simulink model "car_model"  (R2020a)
settings: Solver=FixedStepAuto  StartTime=0.0  StopTime=120  FixedStep=0.01  RelTol=1e-3
values from neighbouring files (symbols this model uses):
  A = 2.18    [car_startup.m]
  brake_force = 7500    [car_startup.m]
  cx = 0.3    [car_startup.m]
  eff = 0.9    [car_startup.m]
  f0 = 0.01    [car_startup.m]
  g = 9.81    [car_startup.m]
  ibi = [3.31 1.91 1.31 0.97 0.81]    [car_startup.m]
  ig = 4.53    [car_startup.m]
  m = 955    [car_startup.m]
  rd = 0.360    (= 0.36)    [car_startup.m]
  start_speed = 0    [car_startup.m]
  torque_curve_f = polyfit(csv_data(:,1), csv_data(:,2), 2)    [car_startup.m]
libraries: simulink x4, SignalEditorBlockLib x1
settings Model: Creator=cp  LastModifiedBy=cp
settings DataIOCC: ReturnWorkspaceOutputs=off  ReturnWorkspaceOutputsName=car
settings OptimizationCC: BlockReduction=off  DefaultParameterBehavior=Inlined  BufferReuse=off

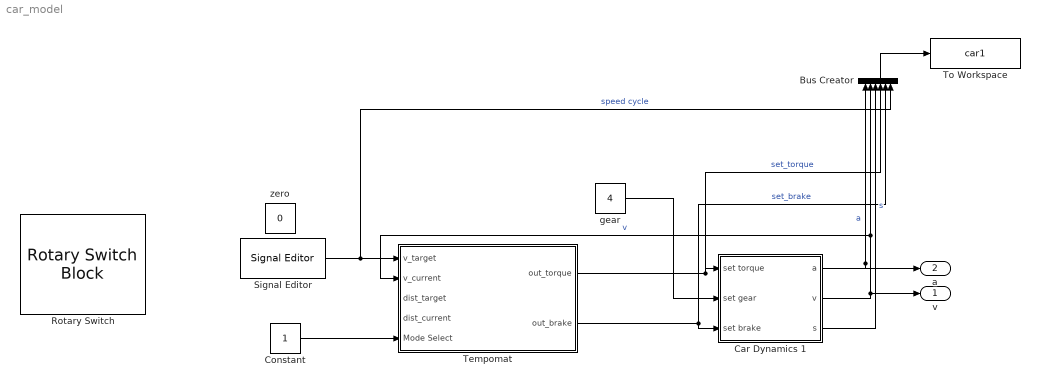
== system car_model ==
  Bus Creator : BusCreator  Inputs=6
  Car Dynamics 1 : Subsystem
  Constant : Constant
  Rotary Switch : RotarySwitchBlock
      settings: Values={{'1', '2', '3', '4', '5'}, [1 2 3 4 5]}
  Signal Editor : SignalEditorBlockLib/Signal Editor  FileName=cycle1.mat  ActiveScenario=Scenario1  ActiveSignal=Signal 1  IsBus=off  OutputBusObjectStr=Bus: BusObject  SampleTime=0  Interpolate=off  ZeroCross=off  OutputAfterFinalValue=Holding final value  Unit=inherit  PreserveSignalName=on
  Tempomat : Subsystem
  To Workspace : ToWorkspace  VariableName=car1  SaveFormat=Timeseries  SampleTime=-1
  gear : Constant  Value=4
  v : Outport
  a : Outport  Port=2
  zero : Constant  IOType=siggen  Value=0
  wires:
  Car Dynamics 1/1(a) -> Bus Creator/1, a/1  "a"
  Car Dynamics 1/2(v) -> Tempomat/2(v_current), Bus Creator/2, v/1  "v"
  Tempomat/1(out_torque) -> Car Dynamics 1/1(set torque), Bus Creator/4  "set_torque"
  gear/1 -> Car Dynamics 1/2(set gear)
  Tempomat/2(out_brake) -> Car Dynamics 1/3(set brake), Bus Creator/5  "set_brake"
  Signal Editor/1 -> Bus Creator/6, Tempomat/1(v_target)  "speed cycle"
  Bus Creator/1 -> To Workspace/1
  Car Dynamics 1/3(s) -> Bus Creator/3  "s"
  Constant/1 -> Tempomat/5(Mode Select)

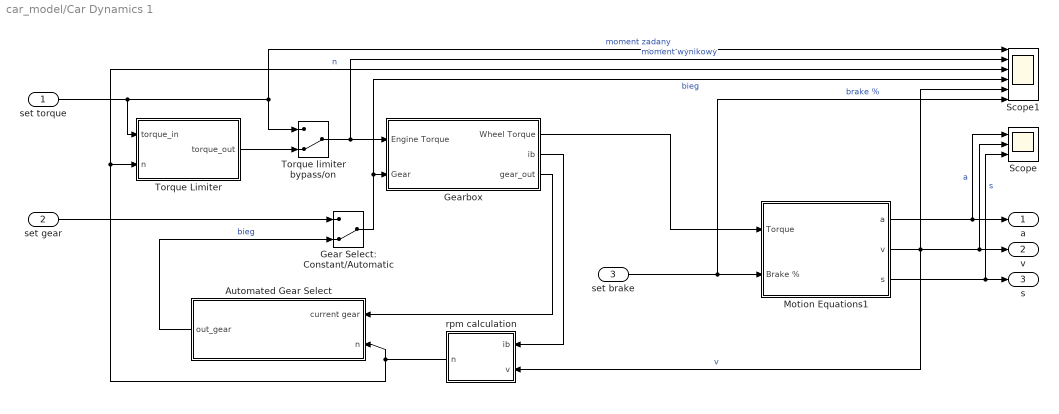
== system car_model/Car Dynamics 1 ==
  set torque : Inport
  set gear : Inport  Port=2
  set brake : Inport  Port=3
  Automated Gear Select : Subsystem
  Gear Select: Constant/Automatic : ManualSwitch  CurrentSetting=0
  Gearbox : Subsystem
  Motion Equations1 : Subsystem  VariantControl=Choice
  Scope : Scope  NumInputPorts=3
  Scope1 : Scope  NumInputPorts=6
  Torque Limiter : Subsystem
  Torque limiter bypass/on : ManualSwitch  CurrentSetting=0
  rpm calculation : Subsystem
  a : Outport
  v : Outport  Port=2
  s : Outport  Port=3
  wires:
  set torque/1 -> Torque limiter bypass/on/1, Scope1/1, Torque Limiter/1(torque_in)  "moment zadany"
  Gearbox/2(ib) -> rpm calculation/1(ib)
  Gear Select: Constant/Automatic/1 -> Scope1/4, Gearbox/2(Gear)  "bieg"
  Automated Gear Select/1(out_gear) -> Gear Select: Constant/Automatic/2  "bieg"
  set gear/1 -> Gear Select: Constant/Automatic/1
  Gearbox/3(gear_out) -> Automated Gear Select/1(current gear)
  rpm calculation/1(n) -> Scope1/3, Torque Limiter/2(n), Automated Gear Select/2(n)  "n"
  Torque limiter bypass/on/1 -> Scope1/2, Gearbox/1(Engine Torque)  "moment wynikowy"
  Torque Limiter/1(torque_out) -> Torque limiter bypass/on/2
  set brake/1 -> Motion Equations1/2(Brake %), Scope1/6  "brake %"
  Gearbox/1(Wheel Torque) -> Motion Equations1/1(Torque)
  Motion Equations1/1(a) -> Scope/1, a/1  "a"
  Motion Equations1/2(v) -> Scope/2, v/1, Scope1/5, rpm calculation/2(v)  "v"
  Motion Equations1/3(s) -> Scope/3, s/1  "s"

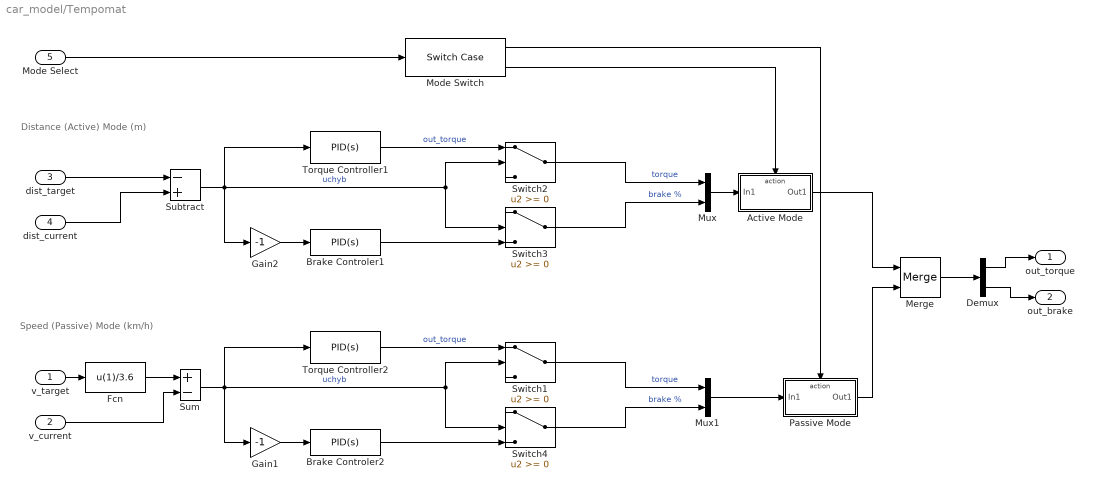
== system car_model/Tempomat ==
  note: Distance (Active) Mode (m)
  note: Speed (Passive) Mode (km/h)
  v_target : Inport
  v_current : Inport  Port=2
  dist_target : Inport  Port=3
  dist_current : Inport  Port=4
  Mode Select : Inport  Port=5
  Active Mode : Subsystem  TreatAsAtomicUnit=on
  Brake Controler1 : simulink/Continuous/PID Controller  Controller=PID  Form=Parallel  TimeDomain=Continuous-time  UseExternalTs=off  SampleTime=-1  IntegratorMethod=Forward Euler  FilterMethod=Forward Euler  ControllerParametersSource=internal  P=5  I=0.5  D=0  UseFilter=on  N=100  TunerSelectOption=Transfer Function Based (PID Tuner App)  InitialConditionSource=internal  InitialConditionForIntegrator=0  InitialConditionForFilter=0  DifferentiatorICPrevScaledInput=0  ExternalReset=none  TrackingMode=off  Kt=1  LimitOutput=on  UpperSaturationLimit=100  LowerSaturationLimit=0  LinearizeAsGain=on  AntiWindupMode=none  Kb=1  POutMin=[]  POutMax=[]  IOutMin=[]  IOutMax=[]  DOutMin=[]  DOutMax=[]  NOutMin=[]  NOutMax=[]  SumOutMin=[]  SumOutMax=[]  SaturationOutMin=[]  SaturationOutMax=[]  PParamMin=[]  PParamMax=[]  IParamMin=[]  IParamMax=[]  DParamMin=[]  DParamMax=[]  NParamMin=[]  NParamMax=[]  KbParamMin=[]  KbParamMax=[]  KtParamMin=[]  KtParamMax=[]  KbOutMin=[]  KbOutMax=[]  KtOutMin=[]  KtOutMax=[]  IntegratorOutMin=[]  IntegratorOutMax=[]  FilterOutMin=[]  FilterOutMax=[]  SumI1OutMin=[]  SumI1OutMax=[]  SumI2OutMin=[]  SumI2OutMax=[]  SumI3OutMin=[]  SumI3OutMax=[]  SumI4OutMin=[]  SumI4OutMax=[]  SumDOutMin=[]  SumDOutMax=[]  DifferentiatorOutMin=[]  DifferentiatorOutMax=[]  FilterDiffOutCoefMin=[]  FilterDiffOutCoefMax=[]  ReciprocalOutMin=[]  ReciprocalOutMax=[]  SumDenOutMin=[]  SumDenOutMax=[]  SumNumOutMin=[]  SumNumOutMax=[]  DivideOutMin=[]  DivideOutMax=[]  UdiffTsProdOutMin=[]  UdiffTsProdOutMax=[]  NTsProdOutMin=[]  NTsProdOutMax=[]  UintegralTsProdOutMin=[]  UintegralTsProdOutMax=[]  UngainTsProdOutMin=[]  UngainTsProdOutMax=[]  IntegratorContinuousStateAttributes=''  IntegratorStateMustResolveToSignalObject=off  IntegratorRTWStateStorageClass=Auto  FilterContinuousStateAttributes=''  FilterStateMustResolveToSignalObject=off  FilterRTWStateStorageClass=Auto  ParallelPVariant=InternalParameters  IdealPVariant=Disabled  IVariant=InternalParameters  DVariant=InternalParameters  IntegratorVariant=Continuous  SatVariant=Enabled  AWVariant=Passthrough  PCopyVariant=Disabled  TRVariant=Disabled  FdbkBlocksVariant=Forward  IdealPFdbkVariant=Disabled  SatFdbkVariant=Disabled  DerivativeFilterVariant=ContFilter  NVariant=InternalParameters  NCopyVariant=Disabled  FilterICVariant=InternalICsFilter  IntegratorICVariant=InternalICs  ExternalResetVariant=Disabled  TRSumVariant=Passthrough  SumFdbkVariant=Disabled  SumVariant=Sum_PID  TsampFilterVariant=InternalTs  TsampNgainVariant=Passthrough  TsampIntegralVariant=Passthrough
  Brake Controler2 : simulink/Continuous/PID Controller  Controller=PID  Form=Parallel  TimeDomain=Continuous-time  UseExternalTs=off  SampleTime=-1  IntegratorMethod=Forward Euler  FilterMethod=Forward Euler  ControllerParametersSource=internal  P=5  I=0.5  D=0  UseFilter=on  N=100  TunerSelectOption=Transfer Function Based (PID Tuner App)  InitialConditionSource=internal  InitialConditionForIntegrator=0  InitialConditionForFilter=0  DifferentiatorICPrevScaledInput=0  ExternalReset=none  TrackingMode=off  Kt=1  LimitOutput=on  UpperSaturationLimit=100  LowerSaturationLimit=0  LinearizeAsGain=on  AntiWindupMode=none  Kb=1  POutMin=[]  POutMax=[]  IOutMin=[]  IOutMax=[]  DOutMin=[]  DOutMax=[]  NOutMin=[]  NOutMax=[]  SumOutMin=[]  SumOutMax=[]  SaturationOutMin=[]  SaturationOutMax=[]  PParamMin=[]  PParamMax=[]  IParamMin=[]  IParamMax=[]  DParamMin=[]  DParamMax=[]  NParamMin=[]  NParamMax=[]  KbParamMin=[]  KbParamMax=[]  KtParamMin=[]  KtParamMax=[]  KbOutMin=[]  KbOutMax=[]  KtOutMin=[]  KtOutMax=[]  IntegratorOutMin=[]  IntegratorOutMax=[]  FilterOutMin=[]  FilterOutMax=[]  SumI1OutMin=[]  SumI1OutMax=[]  SumI2OutMin=[]  SumI2OutMax=[]  SumI3OutMin=[]  SumI3OutMax=[]  SumI4OutMin=[]  SumI4OutMax=[]  SumDOutMin=[]  SumDOutMax=[]  DifferentiatorOutMin=[]  DifferentiatorOutMax=[]  FilterDiffOutCoefMin=[]  FilterDiffOutCoefMax=[]  ReciprocalOutMin=[]  ReciprocalOutMax=[]  SumDenOutMin=[]  SumDenOutMax=[]  SumNumOutMin=[]  SumNumOutMax=[]  DivideOutMin=[]  DivideOutMax=[]  UdiffTsProdOutMin=[]  UdiffTsProdOutMax=[]  NTsProdOutMin=[]  NTsProdOutMax=[]  UintegralTsProdOutMin=[]  UintegralTsProdOutMax=[]  UngainTsProdOutMin=[]  UngainTsProdOutMax=[]  IntegratorContinuousStateAttributes=''  IntegratorStateMustResolveToSignalObject=off  IntegratorRTWStateStorageClass=Auto  FilterContinuousStateAttributes=''  FilterStateMustResolveToSignalObject=off  FilterRTWStateStorageClass=Auto  ParallelPVariant=InternalParameters  IdealPVariant=Disabled  IVariant=InternalParameters  DVariant=InternalParameters  IntegratorVariant=Continuous  SatVariant=Enabled  AWVariant=Passthrough  PCopyVariant=Disabled  TRVariant=Disabled  FdbkBlocksVariant=Forward  IdealPFdbkVariant=Disabled  SatFdbkVariant=Disabled  DerivativeFilterVariant=ContFilter  NVariant=InternalParameters  NCopyVariant=Disabled  FilterICVariant=InternalICsFilter  IntegratorICVariant=InternalICs  ExternalResetVariant=Disabled  TRSumVariant=Passthrough  SumFdbkVariant=Disabled  SumVariant=Sum_PID  TsampFilterVariant=InternalTs  TsampNgainVariant=Passthrough  TsampIntegralVariant=Passthrough
  Demux : Demux  Outputs=2
  Fcn : Fcn  Expr=u(1)/3.6
  Gain1 : Gain  Gain=-1
  Gain2 : Gain  Gain=-1
  Merge : Merge
  Mode Switch : SwitchCase
  Mux : Mux  Inputs=2
  Mux1 : Mux  Inputs=2
  Passive Mode : Subsystem  TreatAsAtomicUnit=on
  Subtract : Sum  Inputs=-+
  Sum : Sum  Inputs=+-
  Switch{1..4} (4 alike) : Switch
  Torque Controller1 : simulink/Continuous/PID Controller  Controller=PID  Form=Parallel  TimeDomain=Continuous-time  UseExternalTs=off  SampleTime=-1  IntegratorMethod=Forward Euler  FilterMethod=Forward Euler  ControllerParametersSource=internal  P=63.1289554713546  I=0  D=0  UseFilter=on  N=0.822866017947126  TunerSelectOption=Transfer Function Based (PID Tuner App)  InitialConditionSource=internal  InitialConditionForIntegrator=0  InitialConditionForFilter=0  DifferentiatorICPrevScaledInput=0  ExternalReset=none  TrackingMode=off  Kt=1  LimitOutput=on  UpperSaturationLimit=148  LowerSaturationLimit=0  LinearizeAsGain=on  AntiWindupMode=none  Kb=1  POutMin=[]  POutMax=[]  IOutMin=[]  IOutMax=[]  DOutMin=[]  DOutMax=[]  NOutMin=[]  NOutMax=[]  SumOutMin=[]  SumOutMax=[]  SaturationOutMin=[]  SaturationOutMax=[]  PParamMin=[]  PParamMax=[]  IParamMin=[]  IParamMax=[]  DParamMin=[]  DParamMax=[]  NParamMin=[]  NParamMax=[]  KbParamMin=[]  KbParamMax=[]  KtParamMin=[]  KtParamMax=[]  KbOutMin=[]  KbOutMax=[]  KtOutMin=[]  KtOutMax=[]  IntegratorOutMin=[]  IntegratorOutMax=[]  FilterOutMin=[]  FilterOutMax=[]  SumI1OutMin=[]  SumI1OutMax=[]  SumI2OutMin=[]  SumI2OutMax=[]  SumI3OutMin=[]  SumI3OutMax=[]  SumI4OutMin=[]  SumI4OutMax=[]  SumDOutMin=[]  SumDOutMax=[]  DifferentiatorOutMin=[]  DifferentiatorOutMax=[]  FilterDiffOutCoefMin=[]  FilterDiffOutCoefMax=[]  ReciprocalOutMin=[]  ReciprocalOutMax=[]  SumDenOutMin=[]  SumDenOutMax=[]  SumNumOutMin=[]  SumNumOutMax=[]  DivideOutMin=[]  DivideOutMax=[]  UdiffTsProdOutMin=[]  UdiffTsProdOutMax=[]  NTsProdOutMin=[]  NTsProdOutMax=[]  UintegralTsProdOutMin=[]  UintegralTsProdOutMax=[]  UngainTsProdOutMin=[]  UngainTsProdOutMax=[]  IntegratorContinuousStateAttributes=''  IntegratorStateMustResolveToSignalObject=off  IntegratorRTWStateStorageClass=Auto  FilterContinuousStateAttributes=''  FilterStateMustResolveToSignalObject=off  FilterRTWStateStorageClass=Auto  ParallelPVariant=InternalParameters  IdealPVariant=Disabled  IVariant=InternalParameters  DVariant=InternalParameters  IntegratorVariant=Continuous  SatVariant=Enabled  AWVariant=Passthrough  PCopyVariant=Disabled  TRVariant=Disabled  FdbkBlocksVariant=Forward  IdealPFdbkVariant=Disabled  SatFdbkVariant=Disabled  DerivativeFilterVariant=ContFilter  NVariant=InternalParameters  NCopyVariant=Disabled  FilterICVariant=InternalICsFilter  IntegratorICVariant=InternalICs  ExternalResetVariant=Disabled  TRSumVariant=Passthrough  SumFdbkVariant=Disabled  SumVariant=Sum_PID  TsampFilterVariant=InternalTs  TsampNgainVariant=Passthrough  TsampIntegralVariant=Passthrough
  Torque Controller2 : simulink/Continuous/PID Controller  Controller=PID  Form=Parallel  TimeDomain=Continuous-time  UseExternalTs=off  SampleTime=-1  IntegratorMethod=Forward Euler  FilterMethod=Forward Euler  ControllerParametersSource=internal  P=63.1289554713546  I=0  D=0  UseFilter=on  N=0.822866017947126  TunerSelectOption=Transfer Function Based (PID Tuner App)  InitialConditionSource=internal  InitialConditionForIntegrator=0  InitialConditionForFilter=0  DifferentiatorICPrevScaledInput=0  ExternalReset=none  TrackingMode=off  Kt=1  LimitOutput=on  UpperSaturationLimit=148  LowerSaturationLimit=0  LinearizeAsGain=on  AntiWindupMode=none  Kb=1  POutMin=[]  POutMax=[]  IOutMin=[]  IOutMax=[]  DOutMin=[]  DOutMax=[]  NOutMin=[]  NOutMax=[]  SumOutMin=[]  SumOutMax=[]  SaturationOutMin=[]  SaturationOutMax=[]  PParamMin=[]  PParamMax=[]  IParamMin=[]  IParamMax=[]  DParamMin=[]  DParamMax=[]  NParamMin=[]  NParamMax=[]  KbParamMin=[]  KbParamMax=[]  KtParamMin=[]  KtParamMax=[]  KbOutMin=[]  KbOutMax=[]  KtOutMin=[]  KtOutMax=[]  IntegratorOutMin=[]  IntegratorOutMax=[]  FilterOutMin=[]  FilterOutMax=[]  SumI1OutMin=[]  SumI1OutMax=[]  SumI2OutMin=[]  SumI2OutMax=[]  SumI3OutMin=[]  SumI3OutMax=[]  SumI4OutMin=[]  SumI4OutMax=[]  SumDOutMin=[]  SumDOutMax=[]  DifferentiatorOutMin=[]  DifferentiatorOutMax=[]  FilterDiffOutCoefMin=[]  FilterDiffOutCoefMax=[]  ReciprocalOutMin=[]  ReciprocalOutMax=[]  SumDenOutMin=[]  SumDenOutMax=[]  SumNumOutMin=[]  SumNumOutMax=[]  DivideOutMin=[]  DivideOutMax=[]  UdiffTsProdOutMin=[]  UdiffTsProdOutMax=[]  NTsProdOutMin=[]  NTsProdOutMax=[]  UintegralTsProdOutMin=[]  UintegralTsProdOutMax=[]  UngainTsProdOutMin=[]  UngainTsProdOutMax=[]  IntegratorContinuousStateAttributes=''  IntegratorStateMustResolveToSignalObject=off  IntegratorRTWStateStorageClass=Auto  FilterContinuousStateAttributes=''  FilterStateMustResolveToSignalObject=off  FilterRTWStateStorageClass=Auto  ParallelPVariant=InternalParameters  IdealPVariant=Disabled  IVariant=InternalParameters  DVariant=InternalParameters  IntegratorVariant=Continuous  SatVariant=Enabled  AWVariant=Passthrough  PCopyVariant=Disabled  TRVariant=Disabled  FdbkBlocksVariant=Forward  IdealPFdbkVariant=Disabled  SatFdbkVariant=Disabled  DerivativeFilterVariant=ContFilter  NVariant=InternalParameters  NCopyVariant=Disabled  FilterICVariant=InternalICsFilter  IntegratorICVariant=InternalICs  ExternalResetVariant=Disabled  TRSumVariant=Passthrough  SumFdbkVariant=Disabled  SumVariant=Sum_PID  TsampFilterVariant=InternalTs  TsampNgainVariant=Passthrough  TsampIntegralVariant=Passthrough
  out_torque : Outport
  out_brake : Outport  Port=2
  wires:
  v_target/1 -> Fcn/1
  Fcn/1 -> Sum/1
  v_current/1 -> Sum/2
  Gain1/1 -> Brake Controler2/1
  Brake Controler2/1 -> Switch4/3
  Switch1/1 -> Mux1/1  "torque"
  Switch4/1 -> Mux1/2  "brake %"
  Torque Controller2/1 -> Switch1/1  "out_torque"
  Sum/1 -> Gain1/1, Switch1/2, Switch4/2, Torque Controller2/1  "uchyb"
  Gain2/1 -> Brake Controler1/1
  Switch3/1 -> Mux/2  "brake %"
  Torque Controller1/1 -> Switch2/1  "out_torque"
  Brake Controler1/1 -> Switch3/3
  Subtract/1 -> Gain2/1, Switch2/2, Switch3/2, Torque Controller1/1  "uchyb"
  Switch2/1 -> Mux/1  "torque"
  Mode Select/1 -> Mode Switch/1
  Mode Switch/2 -> Active Mode/Action
  Mode Switch/1 -> Passive Mode/Action
  Mux/1 -> Active Mode/1(In1)
  Active Mode/1(Out1) -> Merge/1
  Passive Mode/1(Out1) -> Merge/2
  Merge/1 -> Demux/1
  dist_target/1 -> Subtract/1
  dist_current/1 -> Subtract/2
  Demux/1 -> out_torque/1
  Demux/2 -> out_brake/1
  Mux1/1 -> Passive Mode/1(In1)

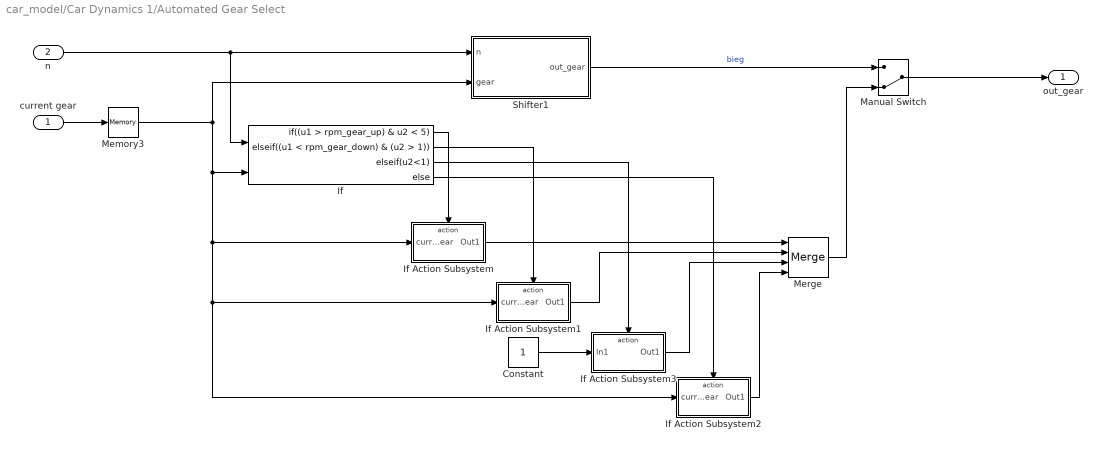
== system car_model/Car Dynamics 1/Automated Gear Select ==
  current gear : Inport
  n : Inport  Port=2
  Constant : Constant
  If : If  NumInputs=2  IfExpression=(u1 > rpm_gear_up) & u2 < 5  ElseIfExpressions=(u1 < rpm_gear_down) & (u2 > 1), u2<1
  If Action Subsystem : Subsystem  TreatAsAtomicUnit=on
  If Action Subsystem1 : Subsystem  TreatAsAtomicUnit=on
  If Action Subsystem2 : Subsystem  TreatAsAtomicUnit=on
  If Action Subsystem3 : Subsystem  TreatAsAtomicUnit=on
  Manual Switch : ManualSwitch  CurrentSetting=0
  Memory3 : Memory
  Merge : Merge  Inputs=4
  Shifter1 : MATLAB Function  TreatAsAtomicUnit=on
  out_gear : Outport
  wires:
  current gear/1 -> Memory3/1
  Memory3/1 -> Shifter1/2(gear), If Action Subsystem2/1(current gear), If Action Subsystem1/1(current gear), If Action Subsystem/1(current gear), If/2
  n/1 -> If/1, Shifter1/1(n)
  If/1 -> If Action Subsystem/Action
  If/2 -> If Action Subsystem1/Action
  If/4 -> If Action Subsystem2/Action
  If Action Subsystem/1(Out1) -> Merge/1
  If Action Subsystem1/1(Out1) -> Merge/2
  If Action Subsystem2/1(Out1) -> Merge/4
  Shifter1/1(out_gear) -> Manual Switch/1  "bieg"
  Manual Switch/1 -> out_gear/1
  Merge/1 -> Manual Switch/2
  If/3 -> If Action Subsystem3/Action
  If Action Subsystem3/1(Out1) -> Merge/3
  Constant/1 -> If Action Subsystem3/1(In1)

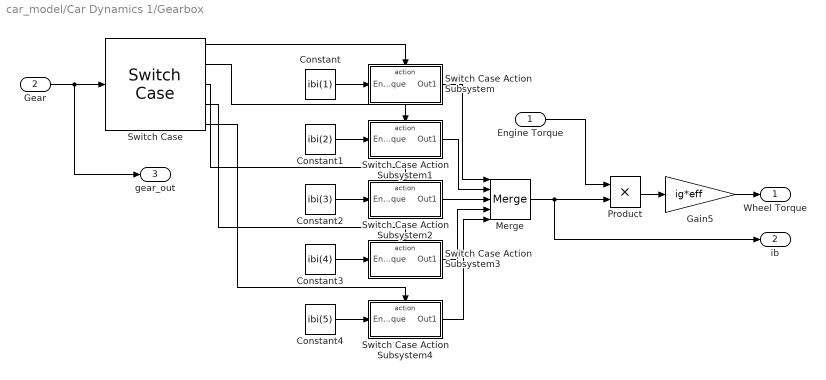
== system car_model/Car Dynamics 1/Gearbox ==
  Engine Torque : Inport
  Gear : Inport  Port=2
  Constant : Constant  Value=ibi(1)
  Constant1 : Constant  Value=ibi(2)
  Constant2 : Constant  Value=ibi(3)
  Constant3 : Constant  Value=ibi(4)
  Constant4 : Constant  Value=ibi(5)
  Gain5 : Gain  Gain=ig*eff
  Merge : Merge  Inputs=5
  Product : Product
  Switch Case : SwitchCase  CaseConditions={[0,1],2,3,4,5}  ShowDefaultCase=off
  Switch Case Action Subsystem : Subsystem  TreatAsAtomicUnit=on
  Switch Case Action Subsystem1 : Subsystem  TreatAsAtomicUnit=on
  Switch Case Action Subsystem2 : Subsystem  TreatAsAtomicUnit=on
  Switch Case Action Subsystem3 : Subsystem  TreatAsAtomicUnit=on
  Switch Case Action Subsystem4 : Subsystem  TreatAsAtomicUnit=on
  Wheel Torque : Outport
  ib : Outport  Port=2
  gear_out : Outport  Port=3
  wires:
  Switch Case/1 -> Switch Case Action Subsystem/Action
  Switch Case/2 -> Switch Case Action Subsystem1/Action
  Switch Case/3 -> Switch Case Action Subsystem2/Action
  Switch Case/4 -> Switch Case Action Subsystem3/Action
  Switch Case/5 -> Switch Case Action Subsystem4/Action
  Constant1/1 -> Switch Case Action Subsystem1/1(Engine Torque)
  Constant/1 -> Switch Case Action Subsystem/1(Engine Torque)
  Switch Case Action Subsystem/1(Out1) -> Merge/1
  Switch Case Action Subsystem1/1(Out1) -> Merge/2
  Switch Case Action Subsystem2/1(Out1) -> Merge/3
  Switch Case Action Subsystem3/1(Out1) -> Merge/4
  Switch Case Action Subsystem4/1(Out1) -> Merge/5
  Gain5/1 -> Wheel Torque/1
  Gear/1 -> gear_out/1, Switch Case/1
  Merge/1 -> ib/1, Product/2
  Product/1 -> Gain5/1
  Engine Torque/1 -> Product/1
  Constant2/1 -> Switch Case Action Subsystem2/1(Engine Torque)
  Constant3/1 -> Switch Case Action Subsystem3/1(Engine Torque)
  Constant4/1 -> Switch Case Action Subsystem4/1(Engine Torque)

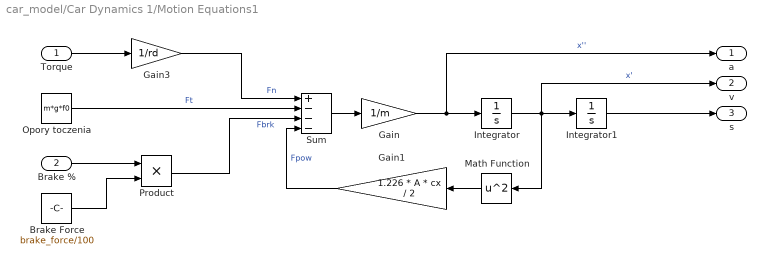
== system car_model/Car Dynamics 1/Motion Equations1 ==
  Torque : Inport
  Brake % : Inport  Port=2
  Brake Force : Constant  Value=brake_force/100
  Gain : Gain  Gain=1/m
  Gain1 : Gain  Gain=1.226 * A * cx / 2
  Gain3 : Gain  Gain=1/rd
  Integrator : Integrator  InitialCondition=start_speed
  Integrator1 : Integrator
  Math Function : Math  Operator=square  SaturateOnIntegerOverflow=on
  Opory toczenia : Constant  Value=m*g*f0
  Product : Product
  Sum : Sum  Inputs=+---
  a : Outport
  v : Outport  Port=2
  s : Outport  Port=3
  wires:
  Integrator1/1 -> s/1
  Sum/1 -> Gain/1
  Math Function/1 -> Gain1/1
  Gain/1 -> a/1, Integrator/1  "x''"
  Integrator/1 -> v/1, Math Function/1, Integrator1/1  "x'"
  Gain1/1 -> Sum/4  "Fpow"
  Opory toczenia/1 -> Sum/2  "Ft"
  Torque/1 -> Gain3/1
  Gain3/1 -> Sum/1  "Fn"
  Brake Force/1 -> Product/2
  Brake %/1 -> Product/1
  Product/1 -> Sum/3  "Fbrk"

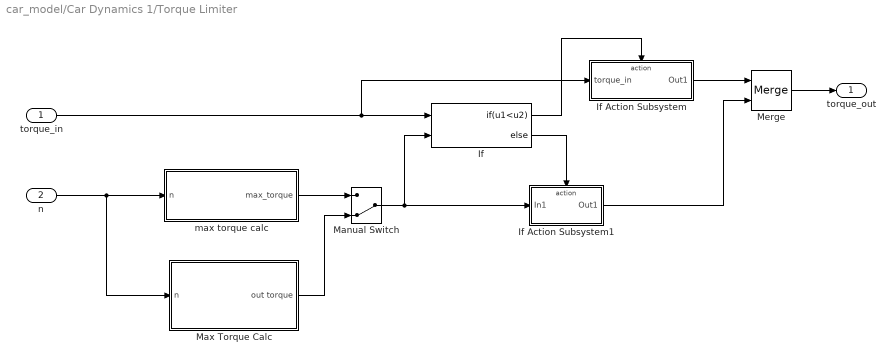
== system car_model/Car Dynamics 1/Torque Limiter ==
  torque_in : Inport
  n : Inport  Port=2
  If : If  NumInputs=2  IfExpression=u1<u2
  If Action Subsystem : Subsystem  TreatAsAtomicUnit=on
  If Action Subsystem1 : Subsystem  TreatAsAtomicUnit=on
  Manual Switch : ManualSwitch  CurrentSetting=0
  Max Torque Calc : Subsystem
  Merge : Merge
  max torque calc : MATLAB Function  TreatAsAtomicUnit=on
  torque_out : Outport
  wires:
  n/1 -> Max Torque Calc/1(n), max torque calc/1(n)
  torque_in/1 -> If Action Subsystem/1(torque_in), If/1
  If/1 -> If Action Subsystem/Action
  Merge/1 -> torque_out/1
  If Action Subsystem/1(Out1) -> Merge/1
  If/2 -> If Action Subsystem1/Action
  If Action Subsystem1/1(Out1) -> Merge/2
  Manual Switch/1 -> If Action Subsystem1/1(In1), If/2
  max torque calc/1(max_torque) -> Manual Switch/1
  Max Torque Calc/1(out torque) -> Manual Switch/2

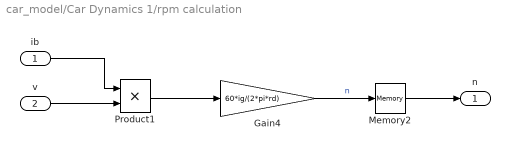
== system car_model/Car Dynamics 1/rpm calculation ==
  ib : Inport
  v : Inport  Port=2
  Gain4 : Gain  Gain=60*ig/(2*pi*rd)
  Memory2 : Memory
  Product1 : Product
  n : Outport
  wires:
  v/1 -> Product1/2
  Memory2/1 -> n/1
  Product1/1 -> Gain4/1
  Gain4/1 -> Memory2/1  "n"
  ib/1 -> Product1/1

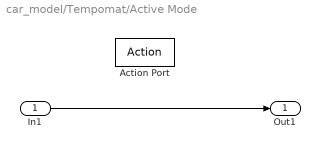
== system car_model/Tempomat/Active Mode ==
  In1 : Inport
  Action Port : ActionPort  ActionPortLabel=default:
  Out1 : Outport
  wires:
  In1/1 -> Out1/1

== system car_model/Tempomat/Passive Mode ==
  In1 : Inport
  Action Port : ActionPort  ActionPortLabel=case [ 1 ]:
  Out1 : Outport
  wires:
  In1/1 -> Out1/1

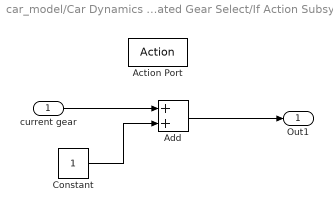
== system car_model/Car Dynamics 1/Automated Gear Select/If Action Subsystem ==
  current gear : Inport
  Action Port : ActionPort  ActionPortLabel=if((u1 > rpm_gear_up) & u2 < 5)
  Add : Sum
  Constant : Constant
  Out1 : Outport
  wires:
  current gear/1 -> Add/1
  Add/1 -> Out1/1
  Constant/1 -> Add/2

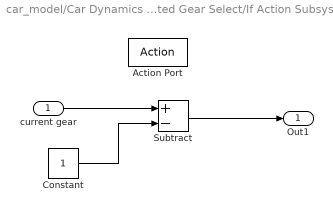
== system car_model/Car Dynamics 1/Automated Gear Select/If Action Subsystem1 ==
  current gear : Inport
  Action Port : ActionPort  ActionPortLabel=elseif((u1 < rpm_gear_down) & (u2 > 1))
  Constant : Constant
  Subtract : Sum  Inputs=+-
  Out1 : Outport
  wires:
  current gear/1 -> Subtract/1
  Subtract/1 -> Out1/1
  Constant/1 -> Subtract/2

== system car_model/Car Dynamics 1/Automated Gear Select/If Action Subsystem2 ==
  current gear : Inport
  Action Port : ActionPort  ActionPortLabel=else
  Out1 : Outport
  wires:
  current gear/1 -> Out1/1

== system car_model/Car Dynamics 1/Automated Gear Select/If Action Subsystem3 ==
  In1 : Inport
  Action Port : ActionPort  ActionPortLabel=elseif( u2<1)
  Out1 : Outport
  wires:
  In1/1 -> Out1/1

== system car_model/Car Dynamics 1/Gearbox/Switch Case Action Subsystem ==
  Engine Torque : Inport
  Action Port : ActionPort  ActionPortLabel=case [ 0 1 ]:
  Out1 : Outport
  wires:
  Engine Torque/1 -> Out1/1

== system car_model/Car Dynamics 1/Gearbox/Switch Case Action Subsystem1 ==
  Engine Torque : Inport
  Action Port : ActionPort  ActionPortLabel=case [ 2 ]:
  Out1 : Outport
  wires:
  Engine Torque/1 -> Out1/1

== system car_model/Car Dynamics 1/Gearbox/Switch Case Action Subsystem2 ==
  Engine Torque : Inport
  Action Port : ActionPort  ActionPortLabel=case [ 3 ]:
  Out1 : Outport
  wires:
  Engine Torque/1 -> Out1/1

== system car_model/Car Dynamics 1/Gearbox/Switch Case Action Subsystem3 ==
  Engine Torque : Inport
  Action Port : ActionPort  ActionPortLabel=case [ 4 ]:
  Out1 : Outport
  wires:
  Engine Torque/1 -> Out1/1

== system car_model/Car Dynamics 1/Gearbox/Switch Case Action Subsystem4 ==
  Engine Torque : Inport
  Action Port : ActionPort  ActionPortLabel=case [ 5 ]:
  Out1 : Outport
  wires:
  Engine Torque/1 -> Out1/1

== system car_model/Car Dynamics 1/Torque Limiter/If Action Subsystem ==
  torque_in : Inport
  Action Port : ActionPort  ActionPortLabel=if(u1<u2)
  Out1 : Outport
  wires:
  torque_in/1 -> Out1/1

== system car_model/Car Dynamics 1/Torque Limiter/If Action Subsystem1 ==
  In1 : Inport
  Action Port : ActionPort  ActionPortLabel=else
  Out1 : Outport
  wires:
  In1/1 -> Out1/1

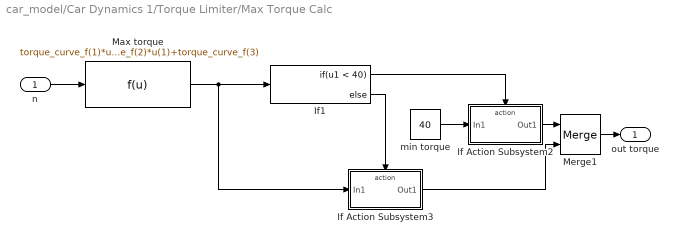
== system car_model/Car Dynamics 1/Torque Limiter/Max Torque Calc ==
  n : Inport
  If Action Subsystem2 : Subsystem  TreatAsAtomicUnit=on
  If Action Subsystem3 : Subsystem  TreatAsAtomicUnit=on
  If1 : If  IfExpression=u1 < 40
  Max torque : Fcn  Expr=torque_curve_f(1)*u(1)^2 + torque_curve_f(2)*u(1)+torque_curve_f(3)
  Merge1 : Merge
  min torque : Constant  Value=40
  out torque : Outport
  wires:
  n/1 -> Max torque/1
  Merge1/1 -> out torque/1
  If Action Subsystem2/1(Out1) -> Merge1/1
  If1/1 -> If Action Subsystem2/Action
  Max torque/1 -> If Action Subsystem3/1(In1), If1/1
  min torque/1 -> If Action Subsystem2/1(In1)
  If Action Subsystem3/1(Out1) -> Merge1/2
  If1/2 -> If Action Subsystem3/Action

== system car_model/Car Dynamics 1/Torque Limiter/Max Torque Calc/If Action Subsystem2 ==
  In1 : Inport
  Action Port : ActionPort  ActionPortLabel=if(u1 < 40)
  Out1 : Outport
  wires:
  In1/1 -> Out1/1

== system car_model/Car Dynamics 1/Torque Limiter/Max Torque Calc/If Action Subsystem3 ==
  In1 : Inport
  Action Port : ActionPort  ActionPortLabel=else
  Out1 : Outport
  wires:
  In1/1 -> Out1/1

== matlab function car_model/Car Dynamics 1/Automated Gear Select/Shifter1 ==
  data: n input; out_gear output; gear input
function out_gear= fcn(n, gear)

if gear < 1
    out_gear = 1;
elseif n > 4500 && gear < 5
    out_gear = gear + 1;
elseif n < 1500 && gear > 1
    out_gear = gear -1;
else
    out_gear = gear;
end

== matlab function car_model/Car Dynamics 1/Torque Limiter/max torque calc ==
  data: n input; max_torque output; torque_curve_f parameter
function max_torque = fcn(n, torque_curve_f)

% oblicz maksymalny dostępny moment na podstawie charakterystyki
% szybkościowej silnika

tmp = polyval(torque_curve_f, n);

if tmp < 40
    max_torque = 40;
else
    max_torque = tmp;
end
